simulink model "c"  (Simulink 9.2)
settings: Solver=VariableStepAuto  StartTime=0.0  StopTime=50  RelTol=1e-3
libraries: fuzblock x1
settings Model: Creator=Administrator  LastModifiedBy=Administrator
settings DataIOCC: LimitDataPoints=off  SaveFormat=Dataset  SignalLoggingSaveFormat=Dataset
settings OptimizationCC: LifeSpan=auto
settings DebuggingCC: UnderspecifiedInitializationDetection=Simplified  MergeDetectMultiDrivingBlocksExec=error  FcnCallInpInsideContextMsg=error  StateNameClashWarn=none  SFUnexpectedBacktrackingDiag=error  SFNoUnconditionalDefaultTransitionDiag=error  SFExecutionAtInitializationDiag=warning
settings HardwareCC: ProdBitPerPointer=64  ProdBitPerSizeT=64  ProdBitPerPtrDiffT=64  ProdLargestAtomicFloat=Float  ProdIntDivRoundTo=Zero  ProdEndianess=LittleEndian  ProdWordSize=64  ProdHWDeviceType=Intel->x86-64 (Windows64)
settings ModelReferenceCC: PropagateSignalLabelsOutOfModel=on
settings SFSimCC: SimUseLocalCustomCode=on
settings RTWCC: RTWUseLocalCustomCode=on
settings CodeAppCC: StateflowObjectComments=off
settings GRTTargetCC: TargetLangStandard=C99 (ISO)  GeneratePreprocessorConditionals=Use local settings  CombineOutputUpdateFcns=on  GRTInterface=off
settings ConfigComp: CovMetricSettings=dwe  CovHtmlReporting=off  CovSaveCumulativeToWorkspaceVar=off  CovSaveSingleToWorkspaceVar=off  CovExternalEMLEnable=on

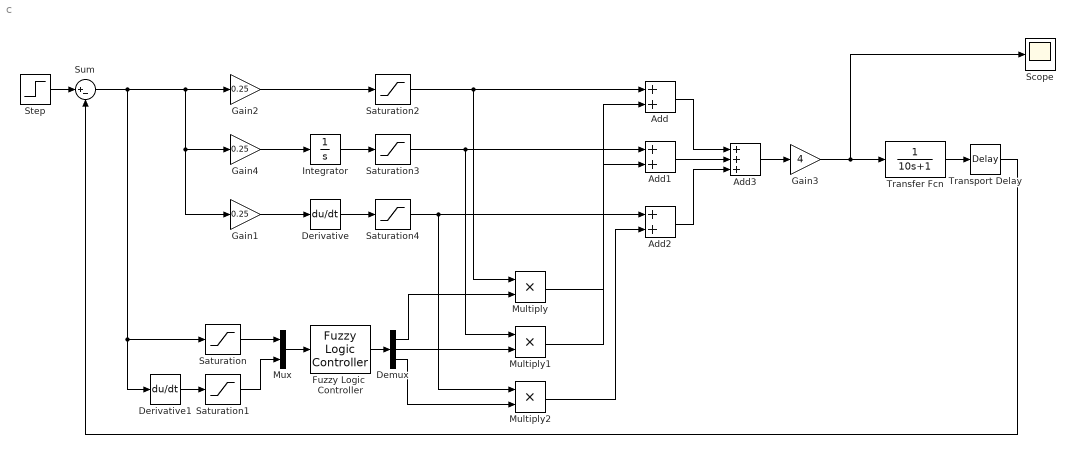
== system c ==
  Add : Sum
  Add1 : Sum
  Add2 : Sum
  Add3 : Sum  Inputs=3
  Demux : Demux  Outputs=3
  Derivative : Derivative
  Derivative1 : Derivative
  Fuzzy Logic  Controller : fuzblock/Fuzzy Logic  Controller  FIS=pid_fuzzy  OutputSampleNumber=101  DataType=double  FuzzifiedInputs=off  RuleFiringStrengths=off  RuleOutputs=off  AggregatedOutputs=off  SimulateUsing=Interpreted execution  OutOfRangeInputValueMessage=warning  NoRuleFiredMessage=warning  EmptyOutputFuzzySetMessage=warning
  Gain1 : Gain  Gain=0.25  SampleTime=0.5
  Gain2 : Gain  Gain=0.25  SampleTime=0.5
  Gain3 : Gain  Gain=4  SampleTime=0.5
  Gain4 : Gain  Gain=0.25  SampleTime=0.5
  Integrator : Integrator
  Multiply : Product
  Multiply1 : Product
  Multiply2 : Product
  Mux : Mux  Inputs=2
  Saturation{,1..4} (5 alike) : Saturate  UpperLimit=3  LowerLimit=-3
  Scope : Scope
  Step : Step  After=30  SampleTime=0
  Sum : Sum  Inputs=|+-
  Transfer Fcn : TransferFcn  Denominator=[10 1]
  Transport Delay : TransportDelay  DelayTime=0.5
  wires:
  Step/1 -> Sum/1
  Transfer Fcn/1 -> Transport Delay/1
  Sum/1 -> Derivative1/1, Saturation/1, Gain2/1, Gain1/1, Gain4/1
  Gain1/1 -> Derivative/1
  Gain4/1 -> Integrator/1
  Gain2/1 -> Saturation2/1
  Integrator/1 -> Saturation3/1
  Derivative/1 -> Saturation4/1
  Multiply/1 -> Add/2
  Multiply1/1 -> Add1/2
  Multiply2/1 -> Add2/2
  Mux/1 -> Fuzzy Logic  Controller/1
  Demux/2 -> Multiply1/2
  Demux/3 -> Multiply2/2
  Demux/1 -> Multiply/2
  Fuzzy Logic  Controller/1 -> Demux/1
  Add/1 -> Add3/1
  Add1/1 -> Add3/2
  Add2/1 -> Add3/3
  Transport Delay/1 -> Sum/2
  Saturation/1 -> Mux/1
  Saturation1/1 -> Mux/2
  Derivative1/1 -> Saturation1/1
  Saturation2/1 -> Multiply/1, Add/1
  Saturation3/1 -> Multiply1/1, Add1/1
  Saturation4/1 -> Multiply2/1, Add2/1
  Add3/1 -> Gain3/1
  Gain3/1 -> Scope/1, Transfer Fcn/1
